simulink model "mariner_sim"  (R2018b)
(part 9 of 22)

      mask Display: e = 0.06;c1 = [120 150 230]/255;c2 = ([120 150 230]+0)/383;c3 = ([120 150 230]+128)/383;patch([0 1 1 0],[0 0 1 1],c1);patch([0 1 1 1-e 1-e 0+e],[0 0 1 1-e 0+e 0+e],c2);patch([0 0 1 1-e 0+e 0+e],[0 1 1 1-e 1-e 0+e],c3);plot([0 1 1 0 0],[0 0 1 1 0]);disp('weights');
  "IW{4,3}(7,:)'" : Constant  Value=[-0.1635846124933579004423478409080416895449161529541015625;-0.162558095028833005102342212921939790248870849609375;0.2013449349190659931618796463226317428052425384521484375;-0.11583555856324799504530886906650266610085964202880859375;-0.0247653101744753911805929647016455419361591339111328125;0.1496170448294603938510505258818739093840122222900390625;-0.267444017975994208224932435769005678594112396240234375;0.11608657921847577443319465828608372248709201812744140625;-0.25854198911053349885236229965812526643276214599609375;-0.1418885172681270956385191084336838684976100921630859375;0.328353020168293152636351805995218455791473388671875;0.02956583414713952195906898623434244655072689056396484375;0.175968715622573601553568778399494476616382598876953125;-0.1861710207919421156130823646890348754823207855224609375;0.287004348529361352770905568831949494779109954833984375;-0.1958607402411904063743719461854198016226291656494140625;0.288637072630618496393850591630325652658939361572265625;-0.12286830490121207482001608468635822646319866180419921875;-0.11186806417272802949280929851738619618117809295654296875;-0.353709703794327701142918840560014359652996063232421875;0.1485319158700189323685236786332097835838794708251953125;0.353481443304769715751945113879628479480743408203125;-0.211414753932288645987824793337495066225528717041015625;0.11530566267047460959904725541491643525660037994384765625;0.020485505610683373001190688000860973261296749114990234375;0.18051592277406403042050442309118807315826416015625;-0.373941353338973769826480975098093040287494659423828125;-0.24093405639050102795550856171757914125919342041015625;0.3631169429600797915469456711434759199619293212890625;-0.2344485351115911664354740651106112636625766754150390625;-0.41789674277581012606930244146496988832950592041015625;0.055755454440739114774228113446952193044126033782958984375;-0.25700915011258940179317278307280503213405609130859375;0.1131734558552566494160629417820018716156482696533203125;0.09474119608271762416062955480811069719493389129638671875;-0.00716245852955323981936519572855104343034327030181884765625;-0.2151817570666623991026966677964082919061183929443359375;-0.12218569917877376840298353499747463501989841461181640625;0.04486655980269622923106709322382812388241291046142578125;0.297034911244270782848531098352395929396152496337890625;0.345689173652893033672484079943387769162654876708984375;-0.1734161524377737517710329484543763101100921630859375;0.158250037536346421784827498413505963981151580810546875;-0.019055729035578526653349484831778681837022304534912109375;-0.2293677944819939862330926416689180769026279449462890625;0.272689515938837667707872469691210426390171051025390625;-0.20232700413925208682286438488517887890338897705078125;-0.340637338023945634990496955651906318962574005126953125]
      mask Display: e = 0.06;c1 = [120 150 230]/255;c2 = ([120 150 230]+0)/383;c3 = ([120 150 230]+128)/383;patch([0 1 1 0],[0 0 1 1],c1);patch([0 1 1 1-e 1-e 0+e],[0 0 1 1-e 0+e 0+e],c2);patch([0 0 1 1-e 0+e 0+e],[0 1 1 1-e 1-e 0+e],c3);plot([0 1 1 0 0],[0 0 1 1 0]);disp('weights');
  "IW{4,3}(8,:)'" : Constant  Value=[0.11018019881404635118560264572806772775948047637939453125;-0.34654832890394315914051048821420408785343170166015625;-0.33275728196639253742006303582456894218921661376953125;-0.35302065620639222487398001248948276042938232421875;-0.100619203604349560787767359215649776160717010498046875;-0.04383868421478930021972786335027194581925868988037109375;-0.251526872104581411537793655952555127441883087158203125;-0.049383110915035895172042756939845276065170764923095703125;-0.048504582443682379977456520236955839209258556365966796875;0.179244900278747565369741323593189008533954620361328125;-0.041547504116541476848478708916445611976087093353271484375;-0.224415646705285409812091756975860334932804107666015625;0.2495143778375682186432271691955975256860256195068359375;0.29179106798029519342918547408771701157093048095703125;0.2176800032431706888313982517502154223620891571044921875;-0.256591581349592645633350684875040315091609954833984375;-0.327988326901448079553347270120866596698760986328125;0.1922294542894002755684113026291015557944774627685546875;0.2680506267551108212643384831608273088932037353515625;-0.059980639853009221074131573914200998842716217041015625;0.221418917140289550626874870431493036448955535888671875;-0.12294895489764291751644265104914666153490543365478515625;-0.1671131502809020952238228119313134811818599700927734375;-0.10534489952314884941841910404036752879619598388671875;0.1799279077362409828833023084371234290301799774169921875;-0.31935807937946159018594016743008978664875030517578125;0.250771027416586023139899452871759422123432159423828125;0.0844867131762666312422282999250455759465694427490234375;0.25698407118216859412740404877695254981517791748046875;-0.170308572534168811696275724898441694676876068115234375;-0.01222357072338942605982392564101246534846723079681396484375;0.1919865858244776124497121827516821213066577911376953125;0.001324566231072940407365035042630552197806537151336669921875;0.28296007629986641429553628768189810216426849365234375;0.343562393621767492302154778371914289891719818115234375;-0.3356757519828625913049791051889769732952117919921875;-0.11509210779102450883382147139855078421533107757568359375;-0.32078925352319098696085575284087099134922027587890625;0.2566614519778769309965582579025067389011383056640625;0.10979171092533672460245242064047488383948802947998046875;0.337822869623220334300839340357924811542034149169921875;-0.0306963793344560663400866218353257863782346248626708984375;0.06557551912767643764734515343661769293248653411865234375;0.2128346310249810413584015122978598810732364654541015625;-0.1356502540548100987916058102200622670352458953857421875;0.280047750033972031591389395543956197798252105712890625;-0.26398238397008111366659477425855584442615509033203125;-0.12212488041810000416464987438303069211542606353759765625]
      mask Display: e = 0.06;c1 = [120 150 230]/255;c2 = ([120 150 230]+0)/383;c3 = ([120 150 230]+128)/383;patch([0 1 1 0],[0 0 1 1],c1);patch([0 1 1 1-e 1-e 0+e],[0 0 1 1-e 0+e 0+e],c2);patch([0 0 1 1-e 0+e 0+e],[0 1 1 1-e 1-e 0+e],c3);plot([0 1 1 0 0],[0 0 1 1 0]);disp('weights');
  "IW{4,3}(9,:)'" : Constant  Value=[-0.33600502309071067497114881916786544024944305419921875;-0.1613131058138488060915705091247218661010265350341796875;-0.154102440400653073471204379529808647930622100830078125;0.275356188971586701708105238139978609979152679443359375;0.26959902262472679179694523554644547402858734130859375;0.12537506787421770493295980486436747014522552490234375;0.07988389945941494485470713016184163279831409454345703125;0.11320765495050590099257448173375451005995273590087890625;0.2377720607906234906447906496396171860396862030029296875;0.140738660577221563752203792319050990045070648193359375;0.0156948978858558914339926815273429383523762226104736328125;-0.368768963689429518648665862201596610248088836669921875;0.355606378493533770157597473371424712240695953369140625;0.1907164031696388095671323981150635518133640289306640625;0.345658937991681958212808467578724958002567291259765625;0.1879492392623798580064686802870710380375385284423828125;-0.1862741822411805581172217216590070165693759918212890625;0.0943651969119596312207676191974314860999584197998046875;-0.095840582171816623979765381591278128325939178466796875;0.2619549498075193216806155760423280298709869384765625;-0.348474552936477000031345596653409302234649658203125;-0.0563632721307514017450301935241441242396831512451171875;0.1341050512561653140775064230183488689363002777099609375;0.1170505153150485921909051967304549179971218109130859375;-0.12290999820828020505647515392411150969564914703369140625;0.049005372112811272644616877869339077733457088470458984375;0.007603282873866687614772263970053245429880917072296142578125;-0.39418086589443646072794535939465276896953582763671875;0.10980423007197841200888177581873605959117412567138671875;0.385307739497387335969591504181153140962123870849609375;-0.322736609179259781310378230045898817479610443115234375;-0.1607908409138828764728401665706769563257694244384765625;-0.2392235725632458065437191407909267581999301910400390625;-0.0782699151547558980013263862929306924343109130859375;-0.0852078763445932307885044565409771166741847991943359375;-0.36404078132169226389436289537115953862667083740234375;-0.2298234704361245828163617943573626689612865447998046875;-0.171423100264454120189583363753627054393291473388671875;-0.1443922039931006262580837073983275331556797027587890625;0.15716622109909217375189882659469731152057647705078125;-0.3720316117009077050425958077539689838886260986328125;0.0581155542518365375581623766265693120658397674560546875;-0.28653839414623882841937074772431515157222747802734375;-0.27136759341804472800419034683727659285068511962890625;0.25788151124619218546030197103391401469707489013671875;-0.0226235331258742185245314004760075476951897144317626953125;-0.07061147677028832558843163269557408057153224945068359375;0.055719126211379206570217803573541459627449512481689453125]
      mask Display: e = 0.06;c1 = [120 150 230]/255;c2 = ([120 150 230]+0)/383;c3 = ([120 150 230]+128)/383;patch([0 1 1 0],[0 0 1 1],c1);patch([0 1 1 1-e 1-e 0+e],[0 0 1 1-e 0+e 0+e],c2);patch([0 0 1 1-e 0+e 0+e],[0 1 1 1-e 1-e 0+e],c3);plot([0 1 1 0 0],[0 0 1 1 0]);disp('weights');
  Mux : Mux  Inputs=48
      mask Display: e = 0.06;c1 = [120 150 230]/255;c2 = ([120 150 230]+0)/383;c3 = ([120 150 230]+128)/383;patch([0 1 1 0],[0 0 1 1],c1);patch([0 1 1 1-e 1-e 0+e],[0 0 1 1-e 0+e 0+e],c2);patch([0 0 1 1-e 0+e 0+e],[0 1 1 1-e 1-e 0+e],c3);plot([0 1 1 0 0],[0 0 1 1 0]);disp('Mux');
  dotprod{1..48} (48 alike) : neural/Weight Functions/dotprod
  "lz{4,3}" : Outport
      mask Display: e = 0.06;c1 = [120 230 180]/255;c2 = ([120 230 180]+0)/(256+128);c3 = ([120 230 180]+128)/(256+128);patch([0 1 1 0],[0 0 1 1],c1);patch([0 1 1 1-e 1-e 0+e],[0 0 1 1-e 0+e 0+e],c2);patch([0 0 1 1-e 0+e 0+e],[0 1 1 1-e 1-e 0+e],c3);plot([0 1 1 0 0],[0 0 1 1 0]);
  wires:
  Mux/1 -> "lz{4,3}"/1
  dotprod48/1 -> Mux/48
  "IW{4,3}(48,:)'"/1 -> dotprod48/1
  dotprod47/1 -> Mux/47
  "IW{4,3}(47,:)'"/1 -> dotprod47/1
  dotprod46/1 -> Mux/46
  "IW{4,3}(46,:)'"/1 -> dotprod46/1
  dotprod45/1 -> Mux/45
  "IW{4,3}(45,:)'"/1 -> dotprod45/1
  dotprod44/1 -> Mux/44
  "IW{4,3}(44,:)'"/1 -> dotprod44/1
  dotprod43/1 -> Mux/43
  "IW{4,3}(43,:)'"/1 -> dotprod43/1
  dotprod42/1 -> Mux/42
  "IW{4,3}(42,:)'"/1 -> dotprod42/1
  dotprod41/1 -> Mux/41
  "IW{4,3}(41,:)'"/1 -> dotprod41/1
  dotprod40/1 -> Mux/40
  "IW{4,3}(40,:)'"/1 -> dotprod40/1
  dotprod39/1 -> Mux/39
  "IW{4,3}(39,:)'"/1 -> dotprod39/1
  dotprod38/1 -> Mux/38
  "IW{4,3}(38,:)'"/1 -> dotprod38/1
  dotprod37/1 -> Mux/37
  "IW{4,3}(37,:)'"/1 -> dotprod37/1
  dotprod36/1 -> Mux/36
  "IW{4,3}(36,:)'"/1 -> dotprod36/1
  dotprod35/1 -> Mux/35
  "IW{4,3}(35,:)'"/1 -> dotprod35/1
  dotprod34/1 -> Mux/34
  "IW{4,3}(34,:)'"/1 -> dotprod34/1
  dotprod33/1 -> Mux/33
  "IW{4,3}(33,:)'"/1 -> dotprod33/1
  dotprod32/1 -> Mux/32
  "IW{4,3}(32,:)'"/1 -> dotprod32/1
  dotprod31/1 -> Mux/31
  "IW{4,3}(31,:)'"/1 -> dotprod31/1
  dotprod30/1 -> Mux/30
  "IW{4,3}(30,:)'"/1 -> dotprod30/1
  dotprod29/1 -> Mux/29
  "IW{4,3}(29,:)'"/1 -> dotprod29/1
  dotprod28/1 -> Mux/28
  "IW{4,3}(28,:)'"/1 -> dotprod28/1
  dotprod27/1 -> Mux/27
  "IW{4,3}(27,:)'"/1 -> dotprod27/1
  dotprod26/1 -> Mux/26
  "IW{4,3}(26,:)'"/1 -> dotprod26/1
  dotprod25/1 -> Mux/25
  "IW{4,3}(25,:)'"/1 -> dotprod25/1
  dotprod24/1 -> Mux/24
  "IW{4,3}(24,:)'"/1 -> dotprod24/1
  dotprod23/1 -> Mux/23
  "IW{4,3}(23,:)'"/1 -> dotprod23/1
  dotprod22/1 -> Mux/22
  "IW{4,3}(22,:)'"/1 -> dotprod22/1
  dotprod21/1 -> Mux/21
  "IW{4,3}(21,:)'"/1 -> dotprod21/1
  dotprod20/1 -> Mux/20
  "IW{4,3}(20,:)'"/1 -> dotprod20/1
  dotprod19/1 -> Mux/19
  "IW{4,3}(19,:)'"/1 -> dotprod19/1
  dotprod18/1 -> Mux/18
  "IW{4,3}(18,:)'"/1 -> dotprod18/1
  dotprod17/1 -> Mux/17
  "IW{4,3}(17,:)'"/1 -> dotprod17/1
  dotprod16/1 -> Mux/16
  "IW{4,3}(16,:)'"/1 -> dotprod16/1
  dotprod15/1 -> Mux/15
  "IW{4,3}(15,:)'"/1 -> dotprod15/1
  dotprod14/1 -> Mux/14
  "IW{4,3}(14,:)'"/1 -> dotprod14/1
  dotprod13/1 -> Mux/13
  "IW{4,3}(13,:)'"/1 -> dotprod13/1
  dotprod12/1 -> Mux/12
  "IW{4,3}(12,:)'"/1 -> dotprod12/1
  dotprod11/1 -> Mux/11
  "IW{4,3}(11,:)'"/1 -> dotprod11/1
  dotprod10/1 -> Mux/10
  "IW{4,3}(10,:)'"/1 -> dotprod10/1
  dotprod9/1 -> Mux/9
  "IW{4,3}(9,:)'"/1 -> dotprod9/1
  dotprod8/1 -> Mux/8
  "IW{4,3}(8,:)'"/1 -> dotprod8/1
  dotprod7/1 -> Mux/7
  "IW{4,3}(7,:)'"/1 -> dotprod7/1
  dotprod6/1 -> Mux/6
  "IW{4,3}(6,:)'"/1 -> dotprod6/1
  dotprod5/1 -> Mux/5
  "IW{4,3}(5,:)'"/1 -> dotprod5/1
  dotprod4/1 -> Mux/4
  "IW{4,3}(4,:)'"/1 -> dotprod4/1
  dotprod3/1 -> Mux/3
  "IW{4,3}(3,:)'"/1 -> dotprod3/1
  dotprod2/1 -> Mux/2
  "IW{4,3}(2,:)'"/1 -> dotprod2/1
  dotprod1/1 -> Mux/1
  "ad{4,3}"/1 -> dotprod48/2, dotprod47/2, dotprod46/2, dotprod45/2, dotprod44/2, dotprod43/2, dotprod42/2, dotprod41/2, dotprod40/2, dotprod39/2, dotprod38/2, dotprod37/2, dotprod36/2, dotprod35/2, dotprod34/2, dotprod33/2, dotprod32/2, dotprod31/2, dotprod30/2, dotprod29/2, dotprod28/2, dotprod27/2, dotprod26/2, dotprod25/2, dotprod24/2, dotprod23/2, dotprod22/2, dotprod21/2, dotprod20/2, dotprod19/2, dotprod18/2, dotprod17/2, dotprod16/2, dotprod15/2, dotprod14/2, dotprod13/2, dotprod12/2, dotprod11/2, dotprod10/2, dotprod9/2, dotprod8/2, dotprod7/2, dotprod6/2, dotprod5/2, dotprod4/2, dotprod3/2, dotprod2/2, dotprod1/2
  "IW{4,3}(1,:)'"/1 -> dotprod1/1
